simulink model "ControlObsSemCanal"  (R2018a)
settings: Solver=VariableStepAuto  StartTime=0.0  StopTime=20.0  RelTol=1e-3
values from neighbouring files (symbols this model uses):
  C = [0.5 1 0]    [ExemploOgata.m]    (also in ProjetoControlPI.m = GYzss.C; dadosLab3.mat = [1 0]; ident.m = GYzss.C)
  F = FKi(1:size(G,2))    [ExemploOgata.m]    (also in ProjetoControlPI.m; dadosLab3.mat = [8860.59286484 122.620823611]; ident.m = acker(G, H, P))
  G = [0 1 0; 0 0 1; -0.12 -0.01 1]    [ExemploOgata.m]    (also in ProjetoControlPI.m = GYzss.A; dadosLab3.mat = [1  0.00945642354217; 0  0.893291168021]; ident.m = GYzss.A)
  H = [0;0;1]    [ExemploOgata.m]    (also in ProjetoControlPI.m = GYzss.B; dadosLab3.mat = [5.749068608e-05 0.0112859265204]; ident.m = GYzss.B)
  Kc = 1/Y(end)    [ExemploOgata.m]    (also in ProjetoControlPI.m; dadosLab3.mat = 0.000112859265204; ident.m = dcgain(SysCtl))
  L = L'    [ProjetoControlPI.m]    (also in dadosLab3.mat = [1.89329116802 84.3838167047]; ident.m)
  Ts = 0.001*fd    (= 0.013)    [ProjetoControlPI.m]    (also in dadosLab3.mat = 0.01; ident.m = 0.01)
settings Model: Creator=castr  LastModifiedBy=castr

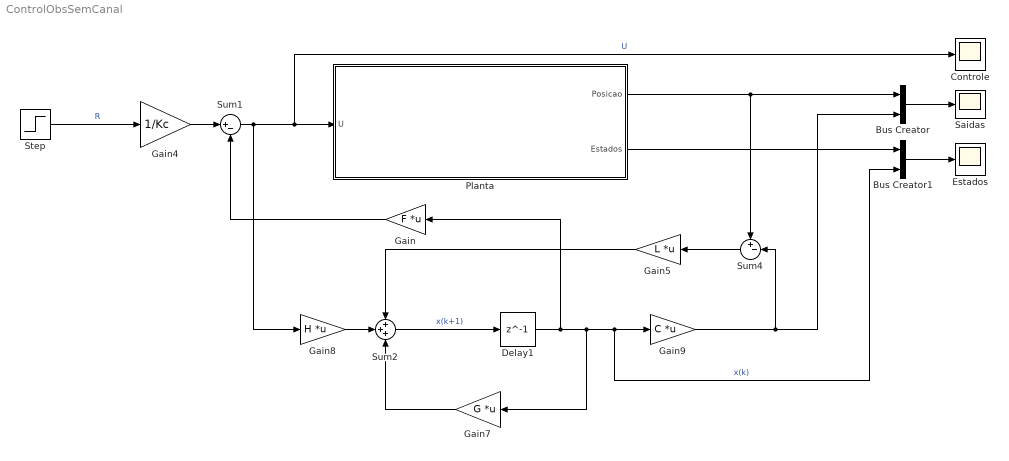
== system ControlObsSemCanal ==
  Bus Creator : BusCreator  Inputs=2
  Bus Creator1 : BusCreator  Inputs=2
  Controle : Scope
  Delay1 : Delay  DelayLength=1  SampleTime=Ts
  Estados : Scope
  Gain : Gain  Gain=F  Multiplication=Matrix(K*u)
  Gain4 : Gain  Gain=1/Kc
  Gain5 : Gain  Gain=L  Multiplication=Matrix(K*u)
  Gain7 : Gain  Gain=G  Multiplication=Matrix(K*u)
  Gain8 : Gain  Gain=H  Multiplication=Matrix(K*u)
  Gain9 : Gain  Gain=C  Multiplication=Matrix(K*u)
  Planta : Subsystem
  Saidas : Scope
  Step : Step  SampleTime=0
  Sum1 : Sum  Inputs=|+-
  Sum2 : Sum  Inputs=+++
  Sum4 : Sum  Inputs=+-|
  wires:
  Sum1/1 -> Gain8/1, Controle/1, Planta/1(U)  "U"
  Gain/1 -> Sum1/2
  Step/1 -> Gain4/1  "R"
  Bus Creator/1 -> Saidas/1
  Sum2/1 -> Delay1/1  "x(k+1)"
  Delay1/1 -> Gain/1, Gain9/1, Bus Creator1/2, Gain7/1  "x(k)"
  Gain4/1 -> Sum1/1
  Gain9/1 -> Sum4/2, Bus Creator/2
  Sum4/1 -> Gain5/1
  Gain7/1 -> Sum2/3
  Gain8/1 -> Sum2/2
  Gain5/1 -> Sum2/1
  Planta/1(Posicao) -> Sum4/1, Bus Creator/1
  Bus Creator1/1 -> Estados/1
  Planta/2(Estados) -> Bus Creator1/1

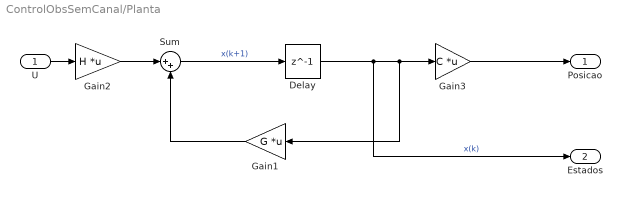
== system ControlObsSemCanal/Planta ==
  U : Inport
  Delay : Delay  DelayLength=1  InitialCondition=[0 0]  SampleTime=Ts
  Gain1 : Gain  Gain=G  Multiplication=Matrix(K*u)
  Gain2 : Gain  Gain=H  Multiplication=Matrix(K*u)
  Gain3 : Gain  Gain=C  Multiplication=Matrix(K*u)
  Sum : Sum  Inputs=|++
  Posicao : Outport
  Estados : Outport  Port=2
  wires:
  Gain1/1 -> Sum/2
  Gain2/1 -> Sum/1
  U/1 -> Gain2/1
  Sum/1 -> Delay/1  "x(k+1)"
  Delay/1 -> Estados/1, Gain1/1, Gain3/1  "x(k)"
  Gain3/1 -> Posicao/1
